simulink model "SimModelV5"  (R2021b)
settings: Solver=FixedStepAuto  StartTime=0.0  StopTime=1200  FixedStep=ts  RelTol=1e-3
InitFcn:
  | simparams
values from neighbouring files (symbols this model uses):
  A_Stirn = 2.19    [simparams.m]
  c_w = 0.25    [simparams.m]
  EngTrq = [0 25 50 75 100 125 150 175 200 225 250 275 300]    [simparams.m]
  f_roll = 0.013    [simparams.m]
  g = 9.81    [simparams.m]
  gear_1 = torque_gear1_excel    [simparams.m]
  Getriebefaktoren = [0.950000000000000	1	1.08000000000000	1.18000000000000	1.26000000000000	1.40000000000000	1.56000000000000	1.13000000000000]    [simparams.m]
  i_brems = 12    [simparams.m]
  i_GetriebeUebersetzung = [0.00, 4.31, 2.44, 1.35, 0.94, 0.82, 0.70, 3.38]    [simparams.m]
  i_UebersetzungHinterachsgetriebe = 3.35    [simparams.m]
  k_Stuetz_Pedal = [0.00 0.13 6.25 12.50 18.75 25.00 31.25 37.50 43.75 50.00 56.25 62.50 68.75 75.00 81.25 90.63 100.00]    [simparams.m]
  m_Fzg = 1525    [simparams.m]
  M_Schlepp = [10.27 10.53 10.93 11.46 12.12 12.91 13.84 14.90 16.09 17.41 18.86 20.45]    [simparams.m]
  m_Zuladung = 50    [simparams.m]
  MassefaktorenGang = [1.04, 1.32, 1.15, 1.10, 1.07, 1.06, 1.05, 1.35]    [simparams.m]
  mu_brems = 0.8    [simparams.m]
  n_brems = 2    [simparams.m]
  n_Stuetz_Motor = [0.00 608.00 640.00 736.00 800.00 992.00 1248.00 1504.00 1760.00 2016.00 2240.00 2496.00 2752.00 3008.00 3264.00 3488.00 3744.00 4000.00 4512.00 4992.00 5248.00 5500.00]    [simparams.m]
  n_Stuetz_Motor_Schlepp = [0 500 1000 1500 2000 2500 3000 3500 4000 4500 5000 5500]    [simparams.m]
  r_brems = 0.1    [simparams.m]
  r_Radradius = 0.32    [simparams.m]
  roh_air = 1.2    [simparams.m]
  torquerequeststandardcondition_pdf = [0 0 0 0 0 0 0 0 0 0 0 0 0 0 0 0 0 0 0 0 0 0 ... (first row only)    [simparams.m]
  U_Radumfang = 2*pi*r_Radradius    (= 2.0106192983)    [simparams.m]
undefined symbols (not defined in the file or in its folder): DiscIntNeverNeededParam
libraries: simulink x2, slpidlib x2
settings Model: Creator=Oli  LastModifiedBy=ruwen
settings DataIOCC: ExternalInput=[cw_drag, A_face, roh_air]

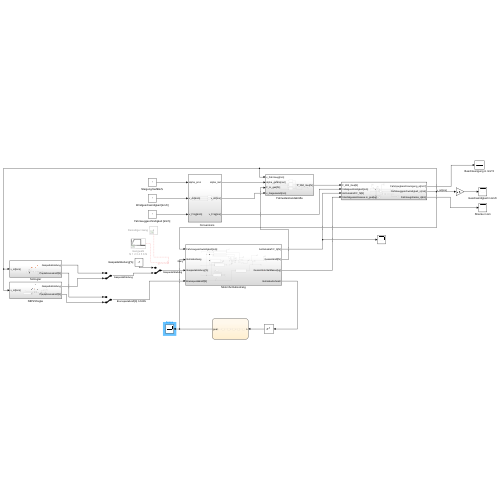
[thumbnail: Simulink's stored preview of the top-level diagram]
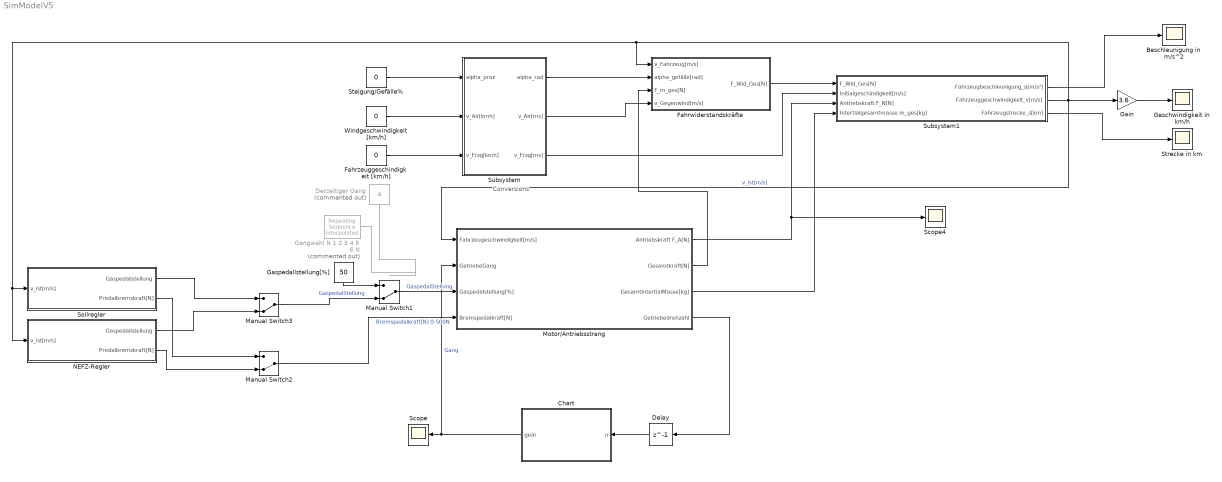
== system SimModelV5 ==
  note: Conversions
  Beschleunigung in m/s^2 : Scope
  Chart : Stateflow chart  TreatAsAtomicUnit=on
  Delay : Delay  DelayLength=1  InitialCondition=0
  Derzeitiger Gang : Constant  Commented=on  Value=4
  Fahrwiderstandskräfte : Subsystem
  Fahrzeuggeschindigkeit [km/h] : Constant  Value=0
  Gain : Gain  Gain=3.6
  Gangwahl N 1 2 3 4 5 6 N : simulink/Sources/Repeating Sequence Interpolated  Commented=on  OutValues="[0   1    2     3    4    5    6     6     0    0].'"  TimeValues=[0 100 200 300 400 500 600 2000 2001 3000].'  LookUpMeth=Use Input Below  tsamp=-1  OutMin=[]  OutMax=[]  OutDataTypeStr=double  OutputDataTypeScalingMode=double  OutDataType=fixdt(0,8)  OutScaling=2^-10
  Gaspedallstellung[%] : Constant  Value=50
  Geschwindigkeit in km/h : Scope
  Manual Switch1 : ManualSwitch  CurrentSetting=0
  Manual Switch2 : ManualSwitch  CurrentSetting=0
  Manual Switch3 : ManualSwitch  CurrentSetting=0
  Motor/Antriebsstrang : Subsystem
  NEFZ-Regler : Subsystem
  Scope : Scope
  Scope4 : Scope
  Sollregler : Subsystem
  "Steigung/Gefälle% " : Constant  Value=0
  Strecke in km : Scope
  Subsystem : Subsystem
  Subsystem1 : Subsystem
  Windgeschwindigkeit [km/h] : Constant  Value=0
  wires:
  "Steigung/Gefälle% "/1 -> Subsystem/1(alpha_proz)
  Windgeschwindigkeit [km/h]/1 -> Subsystem/2(v_Air[kmh])
  Fahrzeuggeschindigkeit [km/h]/1 -> Subsystem/3(v_Frzg[kmh])
  Subsystem/1(alpha_rad) -> Fahrwiderstandskräfte/2(alpha_gefälle[rad])
  Subsystem/2(v_Air[ms]) -> Fahrwiderstandskräfte/4(v_Gegenwind[m/s])
  Fahrwiderstandskräfte/1(F_Wid_Ges[N]) -> Subsystem1/1(F_Wid_Ges[N])
  Subsystem/3(v_Frzg[ms]) -> Subsystem1/2(Initialgeschindigkeit[m/s])
  Motor/Antriebsstrang/3(GesamtIntertialMasse[kg]) -> Subsystem1/4(Intertialgesamtmasse m_ges[kg])
  Motor/Antriebsstrang/2(Gesamtkraft[N]) -> Fahrwiderstandskräfte/3(F_m_ges[N])
  Subsystem1/3(Fahrzeugstrecke_s[km]) -> Strecke in km/1
  Subsystem1/2(Fahrzeuggeschwindigkeit_v[m/s]) -> Gain/1, Motor/Antriebsstrang/1(Fahrzeugeschwindigkeit[m/s]), NEFZ-Regler/1(v_ist[m/s]), Sollregler/1(v_ist[m/s]), Fahrwiderstandskräfte/1(v_Fahrzeug[m/s])  "v_ist[m/s]"
  Subsystem1/1(Fahrzeugbeschleunigung_a[m/s²]) -> Beschleunigung in m/s^2/1
  Derzeitiger Gang/1 -> ?
  Gangwahl N 1 2 3 4 5 6 N/1 -> ?
  Chart/1(gear) -> Motor/Antriebsstrang/2(GetriebeGang), Scope/1  "Gang"
  Gain/1 -> Geschwindigkeit in km/h/1
  Manual Switch1/1 -> Motor/Antriebsstrang/3(Gaspedalstellung[%])  "GaspedalStellung"
  Motor/Antriebsstrang/1(Antriebskraft F_A[N]) -> Subsystem1/3(Antriebskraft F_N[N]), Scope4/1
  Gaspedallstellung[%]/1 -> Manual Switch1/1
  Manual Switch2/1 -> Motor/Antriebsstrang/4(Bremspedalkraft[N])  "Bremspedalkraft[N] 0-500N"
  Manual Switch3/1 -> Manual Switch1/2  "GaspedalStellung"
  NEFZ-Regler/2(Predalbremskraft[N]) -> Manual Switch2/2
  NEFZ-Regler/1(Gaspedallstellung) -> Manual Switch3/2
  Sollregler/1(Gaspedallstellung) -> Manual Switch3/1
  Sollregler/2(Predalbremskraft[N]) -> Manual Switch2/1
  Motor/Antriebsstrang/4(Getriebedrehzahl) -> Delay/1
  Delay/1 -> Chart/1(n)

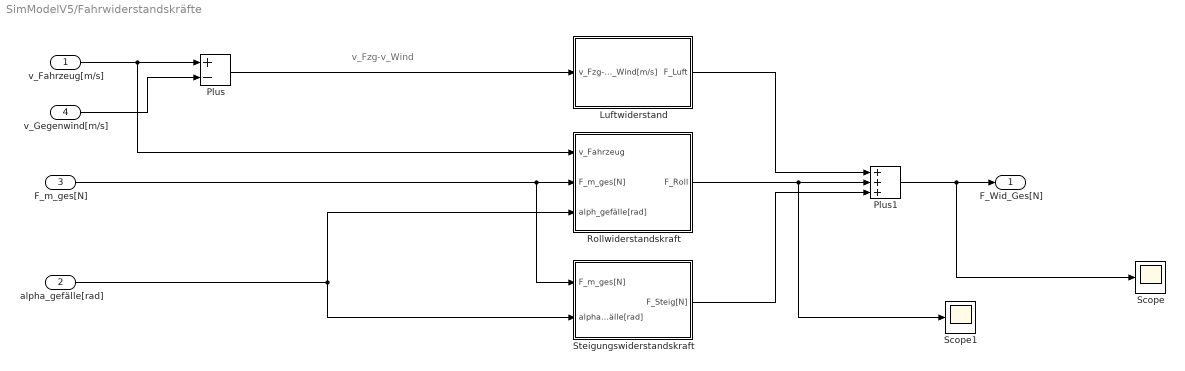
== system SimModelV5/Fahrwiderstandskräfte ==
  note: v_Fzg-v_Wind
  v_Fahrzeug[m/s] : Inport
  alpha_gefälle[rad] : Inport  Port=2
  F_m_ges[N] : Inport  Port=3
  v_Gegenwind[m/s] : Inport  Port=4
  Luftwiderstand : Subsystem
  Plus : Sum  Inputs=+-
  Plus1 : Sum  Inputs=+++
  Rollwiderstandskraft : Subsystem
  Scope : Scope
  Scope1 : Scope
  Steigungswiderstandskraft : Subsystem
  F_Wid_Ges[N] : Outport
  wires:
  v_Fahrzeug[m/s]/1 -> Rollwiderstandskraft/1(v_Fahrzeug), Plus/1
  v_Gegenwind[m/s]/1 -> Plus/2
  Plus/1 -> Luftwiderstand/1(v_Fzg-v_Wind[m/s])
  F_m_ges[N]/1 -> Steigungswiderstandskraft/1(F_m_ges[N]), Rollwiderstandskraft/2(F_m_ges[N])
  alpha_gefälle[rad]/1 -> Steigungswiderstandskraft/2(alpha_gefälle[rad]), Rollwiderstandskraft/3(alph_gefälle[rad])
  Luftwiderstand/1(F_Luft) -> Plus1/1
  Rollwiderstandskraft/1(F_Roll) -> Scope1/1, Plus1/2
  Steigungswiderstandskraft/1(F_Steig[N]) -> Plus1/3
  Plus1/1 -> F_Wid_Ges[N]/1, Scope/1

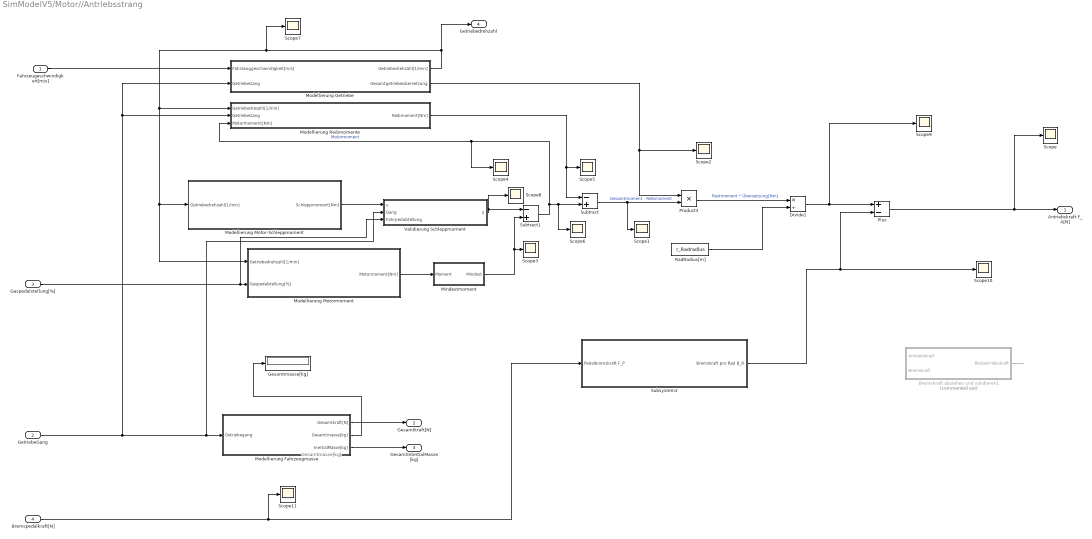
== system SimModelV5/Motor//Antriebsstrang ==
  note: Gesamtmasse[kg]
  Fahrzeugeschwindigkeit[m/s] : Inport
  GetriebeGang : Inport  Port=2
  Gaspedalstellung[%] : Inport  Port=3
  Bremspedalkraft[N] : Inport  Port=4
  Bremskraft abziehen und validieren1 : MATLAB Function  Commented=on  TreatAsAtomicUnit=on
  Divide1 : Product  Inputs=*/
  Gesamtmasse[kg] : Display
  Mindestmoment : Subsystem
  Modellierung Fahrzeugmasse : Subsystem
  Modellierung Getriebe : Subsystem
  Modellierung Motor-Schleppmoment : Subsystem
  Modellierung Motormoment : Subsystem
  Modellierung Reibmomente : Subsystem
  Plus : Sum  Inputs=+-
  Product3 : Product
  RadRadius[m] : Constant  Value=r_Radradius
  Scope{,1..11} (12 alike) : Scope
  Subsystem2 : Subsystem
  Subtract : Sum  Inputs=-+
  Subtract1 : Sum  Inputs=-+
  Validierung Schleppmoment : MATLAB Function  TreatAsAtomicUnit=on
  Antriebskraft F_A[N] : Outport
  Gesamtkraft[N] : Outport  Port=2
  GesamtIntertialMasse[kg] : Outport  Port=3
  Getriebedrehzahl : Outport  Port=4
  wires:
  GetriebeGang/1 -> Modellierung Fahrzeugmasse/1(Getriebegang), Validierung Schleppmoment/2(Gang), Modellierung Reibmomente/2(GetriebeGang), Modellierung Getriebe/2(GetriebeGang)
  Modellierung Fahrzeugmasse/1(Gesamtkraft[N]) -> Gesamtkraft[N]/1
  Modellierung Fahrzeugmasse/2(Gesamtmasse[kg]) -> Gesamtmasse[kg]/1
  Modellierung Fahrzeugmasse/3(InertialMasse[kg]) -> GesamtIntertialMasse[kg]/1
  Modellierung Getriebe/1(Getriebedrehzahl[1/min]) -> Getriebedrehzahl/1, Scope7/1, Modellierung Reibmomente/1(Getriebedrezahl[1/min]), Modellierung Motormoment/1(Getriebedrehzahl[1/min]), Modellierung Motor-Schleppmoment/1(Getriebedrehzahl[1/min])
  Fahrzeugeschwindigkeit[m/s]/1 -> Modellierung Getriebe/1(Fahrzeuggeschwindigkeit[m/s])
  Gaspedalstellung[%]/1 -> Modellierung Motormoment/2(Gaspedalstellung[%]), Validierung Schleppmoment/3(Fahrpedalstellung)
  Modellierung Motor-Schleppmoment/1(Schleppmoment[Nm]) -> Validierung Schleppmoment/1(u)
  Validierung Schleppmoment/1(y) -> Scope8/1, Subtract1/1
  Mindestmoment/1(Mindest) -> Subtract1/2, Scope3/1
  Modellierung Motormoment/1(Motormoment[Nm]) -> Mindestmoment/1(Moment)
  Subtract1/1 -> Scope6/1, Subtract/2, Scope4/1, Modellierung Reibmomente/3(Motormomemt[Nm])  "Motormoment"
  Modellierung Reibmomente/1(Reibmoment[Nm]) -> Scope5/1, Subtract/1
  Subtract/1 -> Scope1/1, Product3/2  "Gesamtmoment - Reibmoment"
  Modellierung Getriebe/2(Gesamtgetriebeübersetzung) -> Scope2/1, Product3/1
  Product3/1 -> Divide1/1  "Restmoment * Übersetzung[Nm]"
  RadRadius[m]/1 -> Divide1/2
  Divide1/1 -> Plus/1, Scope9/1
  Subsystem2/1(Bremskraft pro Rad B_R) -> Plus/2, Scope10/1
  Bremspedalkraft[N]/1 -> Scope11/1, Subsystem2/1(Pedalbremskraft F_P)
  Plus/1 -> Antriebskraft F_A[N]/1, Scope/1
  Bremskraft abziehen und validieren1/1(Restantriebskraft) -> ?

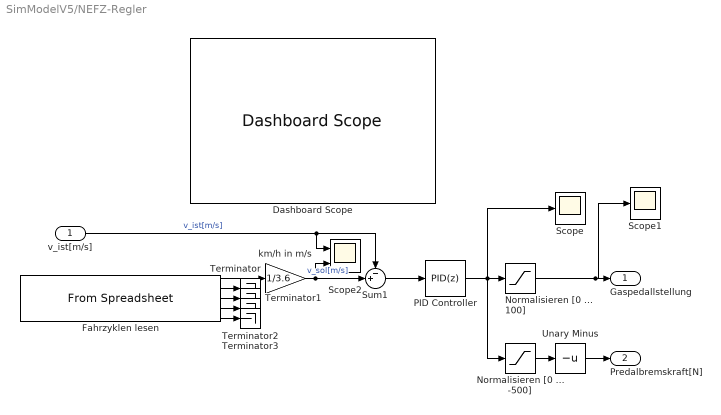
== system SimModelV5/NEFZ-Regler ==
  v_ist[m/s] : Inport
  Dashboard Scope : DashboardScope
  Fahrzyklen lesen : FromSpreadsheet  FileName=Fahrzyklen_Uebung_05.xlsx  SheetName=Tabelle1
  Normalisieren [0 ... -500] : Saturate  UpperLimit=0  LowerLimit=-500
  Normalisieren [0 ... 100] : Saturate  UpperLimit=100  LowerLimit=0
  PID Controller : slpidlib/PID Controller  Controller=PID  Form=Parallel  TimeDomain=Discrete-time  UseExternalTs=off  SampleTime=-1  IntegratorMethod=Forward Euler  FilterMethod=Forward Euler  ControllerParametersSource=internal  P=5000  I=0.78  D=0  UseFilter=on  N=100  TunerSelectOption=Transfer Function Based (PID Tuner App)  InitialConditionSource=internal  InitialConditionForIntegrator=0  InitialConditionForFilter=0  DifferentiatorICPrevScaledInput=0  ExternalReset=none  TrackingMode=off  Kt=1  LimitOutput=off  SatLimitsSource=internal  UpperSaturationLimit=inf  LowerSaturationLimit=-inf  LinearizeAsGain=on  AntiWindupMode=none  Kb=1  POutMin=[]  POutMax=[]  IOutMin=[]  IOutMax=[]  DOutMin=[]  DOutMax=[]  NOutMin=[]  NOutMax=[]  SumOutMin=[]  SumOutMax=[]  SaturationOutMin=[]  SaturationOutMax=[]  PParamMin=[]  PParamMax=[]  IParamMin=[]  IParamMax=[]  DParamMin=[]  DParamMax=[]  NParamMin=[]  NParamMax=[]  KbParamMin=[]  KbParamMax=[]  KtParamMin=[]  KtParamMax=[]  KbOutMin=[]  KbOutMax=[]  KtOutMin=[]  KtOutMax=[]  IntegratorOutMin=[]  IntegratorOutMax=[]  FilterOutMin=[]  FilterOutMax=[]  SumI1OutMin=[]  SumI1OutMax=[]  SumI2OutMin=[]  SumI2OutMax=[]  SumI3OutMin=[]  SumI3OutMax=[]  SumI4OutMin=[]  SumI4OutMax=[]  SumDOutMin=[]  SumDOutMax=[]  DifferentiatorOutMin=[]  DifferentiatorOutMax=[]  FilterDiffOutCoefMin=[]  FilterDiffOutCoefMax=[]  ReciprocalOutMin=[]  ReciprocalOutMax=[]  SumDenOutMin=[]  SumDenOutMax=[]  SumNumOutMin=[]  SumNumOutMax=[]  DivideOutMin=[]  DivideOutMax=[]  UdiffTsProdOutMin=[]  UdiffTsProdOutMax=[]  NTsProdOutMin=[]  NTsProdOutMax=[]  UintegralTsProdOutMin=[]  UintegralTsProdOutMax=[]  UngainTsProdOutMin=[]  UngainTsProdOutMax=[]  IntegratorContinuousStateAttributes=''  IntegratorStateMustResolveToSignalObject=off  IntegratorRTWStateStorageClass=Auto  FilterContinuousStateAttributes=''  FilterStateMustResolveToSignalObject=off  FilterRTWStateStorageClass=Auto  ParallelPVariant=InternalParameters  IdealPVariant=Disabled  IVariant=InternalParameters  DVariant=InternalParameters  IntegratorVariant=Discrete  SatVariant=Disabled  AWVariant=Passthrough  PCopyVariant=Disabled  TRVariant=Disabled  FdbkBlocksVariant=Forward  IdealPFdbkVariant=Disabled  SatFdbkVariant=Disabled  DerivativeFilterVariant=ForwardEulerFilter  NVariant=InternalParameters  NCopyVariant=Disabled  FilterICVariant=InternalICsFilter  IntegratorICVariant=InternalICs  ExternalResetVariant=Disabled  TRSumVariant=Passthrough  SumFdbkVariant=Disabled  SumVariant=Sum_PID  TsampFilterVariant=InternalTs  TsampNgainVariant=Passthrough  TsampIntegralVariant=Passthrough  ExternalSaturationOutDataTypeStr=Inherit: Same as second input
  Scope : Scope
  Scope1 : Scope
  Scope2 : Scope  NumInputPorts=2
  Sum1 : Sum  Inputs=-+|
  Terminator{,1..3} (4 alike) : Terminator
  Unary Minus : UnaryMinus
  km/h in m/s : Gain  Gain=1/3.6
  Gaspedallstellung : Outport
  Predalbremskraft[N] : Outport  Port=2
  wires:
  km/h in m/s/1 -> Sum1/2, Scope2/2  "v_sol[m/s]"
  Sum1/1 -> PID Controller/1
  v_ist[m/s]/1 -> Scope2/1, Sum1/1  "v_ist[m/s]"
  PID Controller/1 -> Scope/1, Normalisieren [0 ... -500]/1, Normalisieren [0 ... 100]/1
  Normalisieren [0 ... 100]/1 -> Scope1/1, Gaspedallstellung/1
  Fahrzyklen lesen/2 -> Terminator/1
  Fahrzyklen lesen/3 -> Terminator1/1
  Fahrzyklen lesen/4 -> Terminator2/1
  Fahrzyklen lesen/5 -> Terminator3/1
  Fahrzyklen lesen/1 -> km/h in m/s/1
  Normalisieren [0 ... -500]/1 -> Unary Minus/1
  Unary Minus/1 -> Predalbremskraft[N]/1

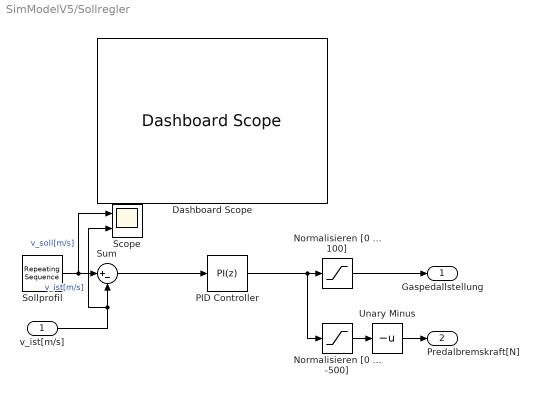
== system SimModelV5/Sollregler ==
  v_ist[m/s] : Inport
  Dashboard Scope : DashboardScope
  Normalisieren [0 ... -500] : Saturate  UpperLimit=0  LowerLimit=-500
  Normalisieren [0 ... 100] : Saturate  UpperLimit=100  LowerLimit=0
  PID Controller : slpidlib/PID Controller  Controller=PI  Form=Parallel  TimeDomain=Discrete-time  UseExternalTs=off  SampleTime=-1  IntegratorMethod=Forward Euler  FilterMethod=Forward Euler  ControllerParametersSource=internal  P=25  I=1  D=-1  UseFilter=on  N=100  TunerSelectOption=Transfer Function Based (PID Tuner App)  InitialConditionSource=internal  InitialConditionForIntegrator=0  InitialConditionForFilter=0  DifferentiatorICPrevScaledInput=0  ExternalReset=none  TrackingMode=off  Kt=1  LimitOutput=off  SatLimitsSource=internal  UpperSaturationLimit=inf  LowerSaturationLimit=-inf  LinearizeAsGain=on  AntiWindupMode=none  Kb=1  POutMin=[]  POutMax=[]  IOutMin=[]  IOutMax=[]  DOutMin=[]  DOutMax=[]  NOutMin=[]  NOutMax=[]  SumOutMin=[]  SumOutMax=[]  SaturationOutMin=[]  SaturationOutMax=[]  PParamMin=[]  PParamMax=[]  IParamMin=[]  IParamMax=[]  DParamMin=[]  DParamMax=[]  NParamMin=[]  NParamMax=[]  KbParamMin=[]  KbParamMax=[]  KtParamMin=[]  KtParamMax=[]  KbOutMin=[]  KbOutMax=[]  KtOutMin=[]  KtOutMax=[]  IntegratorOutMin=[]  IntegratorOutMax=[]  FilterOutMin=[]  FilterOutMax=[]  SumI1OutMin=[]  SumI1OutMax=[]  SumI2OutMin=[]  SumI2OutMax=[]  SumI3OutMin=[]  SumI3OutMax=[]  SumI4OutMin=[]  SumI4OutMax=[]  SumDOutMin=[]  SumDOutMax=[]  DifferentiatorOutMin=[]  DifferentiatorOutMax=[]  FilterDiffOutCoefMin=[]  FilterDiffOutCoefMax=[]  ReciprocalOutMin=[]  ReciprocalOutMax=[]  SumDenOutMin=[]  SumDenOutMax=[]  SumNumOutMin=[]  SumNumOutMax=[]  DivideOutMin=[]  DivideOutMax=[]  UdiffTsProdOutMin=[]  UdiffTsProdOutMax=[]  NTsProdOutMin=[]  NTsProdOutMax=[]  UintegralTsProdOutMin=[]  UintegralTsProdOutMax=[]  UngainTsProdOutMin=[]  UngainTsProdOutMax=[]  IntegratorContinuousStateAttributes=''  IntegratorStateMustResolveToSignalObject=off  IntegratorRTWStateStorageClass=Auto  FilterContinuousStateAttributes=''  FilterStateMustResolveToSignalObject=off  FilterRTWStateStorageClass=Auto  ParallelPVariant=InternalParameters  IdealPVariant=Disabled  IVariant=InternalParameters  DVariant=Disabled  IntegratorVariant=Discrete  SatVariant=Disabled  AWVariant=Passthrough  PCopyVariant=Disabled  TRVariant=Disabled  FdbkBlocksVariant=Forward  IdealPFdbkVariant=Disabled  SatFdbkVariant=Disabled  DerivativeFilterVariant=Disabled  NVariant=Disabled  NCopyVariant=Disabled_SignalSpec  FilterICVariant=Disabled  IntegratorICVariant=InternalICs  ExternalResetVariant=Disabled  TRSumVariant=Passthrough  SumFdbkVariant=Disabled  SumVariant=Sum_PI  TsampFilterVariant=InternalTs  TsampNgainVariant=Passthrough  TsampIntegralVariant=Passthrough  ExternalSaturationOutDataTypeStr=Inherit: Same as second input
  Scope : Scope  NumInputPorts=2
  Sollprofil : simulink/Sources/Repeating Sequence  rep_seq_t=[0 50 100 1100 1150 1200]  rep_seq_y=[0 0 27 44 0 0]
  Sum : Sum  Inputs=|+-
  Unary Minus : UnaryMinus
  Gaspedallstellung : Outport
  Predalbremskraft[N] : Outport  Port=2
  wires:
  Sollprofil/1 -> Scope/1, Sum/1  "v_soll[m/s]"
  v_ist[m/s]/1 -> Scope/2, Sum/2  "v_ist[m/s]"
  PID Controller/1 -> Normalisieren [0 ... -500]/1, Normalisieren [0 ... 100]/1
  Normalisieren [0 ... 100]/1 -> Gaspedallstellung/1
  Sum/1 -> PID Controller/1
  Normalisieren [0 ... -500]/1 -> Unary Minus/1
  Unary Minus/1 -> Predalbremskraft[N]/1

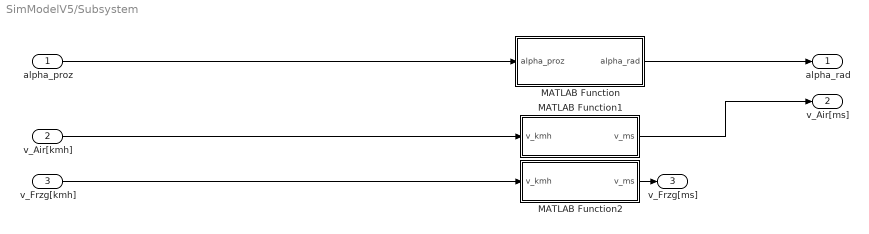
== system SimModelV5/Subsystem ==
  alpha_proz : Inport
  v_Air[kmh] : Inport  Port=2
  v_Frzg[kmh] : Inport  Port=3
  MATLAB Function : MATLAB Function  TreatAsAtomicUnit=on
  MATLAB Function1 : MATLAB Function  TreatAsAtomicUnit=on
  MATLAB Function2 : MATLAB Function  TreatAsAtomicUnit=on
  alpha_rad : Outport
  v_Air[ms] : Outport  Port=2
  v_Frzg[ms] : Outport  Port=3
  wires:
  v_Frzg[kmh]/1 -> MATLAB Function2/1(v_kmh)
  MATLAB Function/1(alpha_rad) -> alpha_rad/1
  alpha_proz/1 -> MATLAB Function/1(alpha_proz)
  MATLAB Function2/1(v_ms) -> v_Frzg[ms]/1
  v_Air[kmh]/1 -> MATLAB Function1/1(v_kmh)
  MATLAB Function1/1(v_ms) -> v_Air[ms]/1

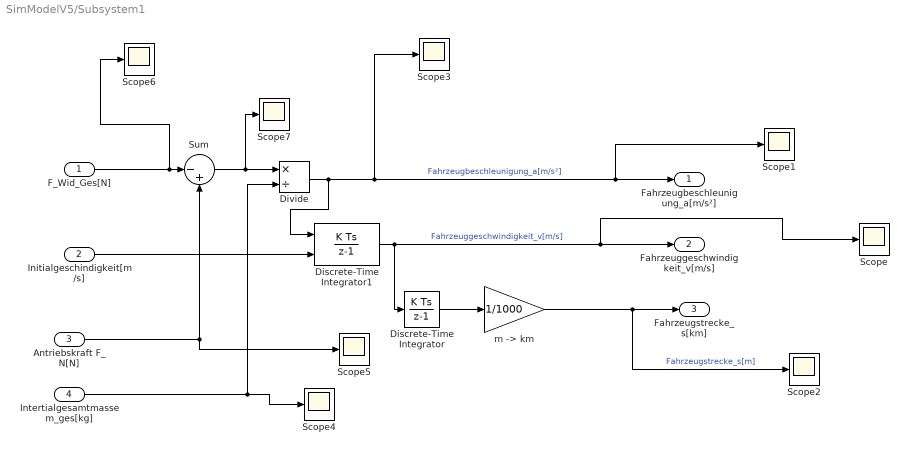
== system SimModelV5/Subsystem1 ==
  F_Wid_Ges[N] : Inport
  Initialgeschindigkeit[m/s] : Inport  Port=2
  Antriebskraft F_N[N] : Inport  Port=3
  Intertialgesamtmasse m_ges[kg] : Inport  Port=4
  Discrete-Time Integrator : DiscreteIntegrator  SampleTime=-1  ICPrevOutput=DiscIntNeverNeededParam  ICPrevScaledInput=DiscIntNeverNeededParam
  Discrete-Time Integrator1 : DiscreteIntegrator  InitialConditionSource=external  SampleTime=-1  LimitOutput=on  UpperSaturationLimit=100  ICPrevOutput=DiscIntNeverNeededParam  ICPrevScaledInput=DiscIntNeverNeededParam
  Divide : Product  Inputs=*/
  Scope{,1..7} (8 alike) : Scope
  Sum : Sum  Inputs=|-+
  "m -> km" : Gain  Gain=1/1000
  Fahrzeugbeschleunigung_a[m/s²] : Outport
  Fahrzeuggeschwindigkeit_v[m/s] : Outport  Port=2
  Fahrzeugstrecke_s[km] : Outport  Port=3
  wires:
  Sum/1 -> Scope7/1, Divide/1
  "m -> km"/1 -> Scope2/1, Fahrzeugstrecke_s[km]/1  "Fahrzeugstrecke_s[m]"
  Divide/1 -> Discrete-Time Integrator1/1, Scope3/1, Scope1/1, Fahrzeugbeschleunigung_a[m/s²]/1  "Fahrzeugbeschleunigung_a[m/s²]"
  Discrete-Time Integrator/1 -> "m -> km"/1
  Intertialgesamtmasse m_ges[kg]/1 -> Scope4/1, Divide/2
  F_Wid_Ges[N]/1 -> Scope6/1, Sum/1
  Discrete-Time Integrator1/1 -> Discrete-Time Integrator/1, Scope/1, Fahrzeuggeschwindigkeit_v[m/s]/1  "Fahrzeuggeschwindigkeit_v[m/s]"
  Antriebskraft F_N[N]/1 -> Scope5/1, Sum/2
  Initialgeschindigkeit[m/s]/1 -> Discrete-Time Integrator1/2

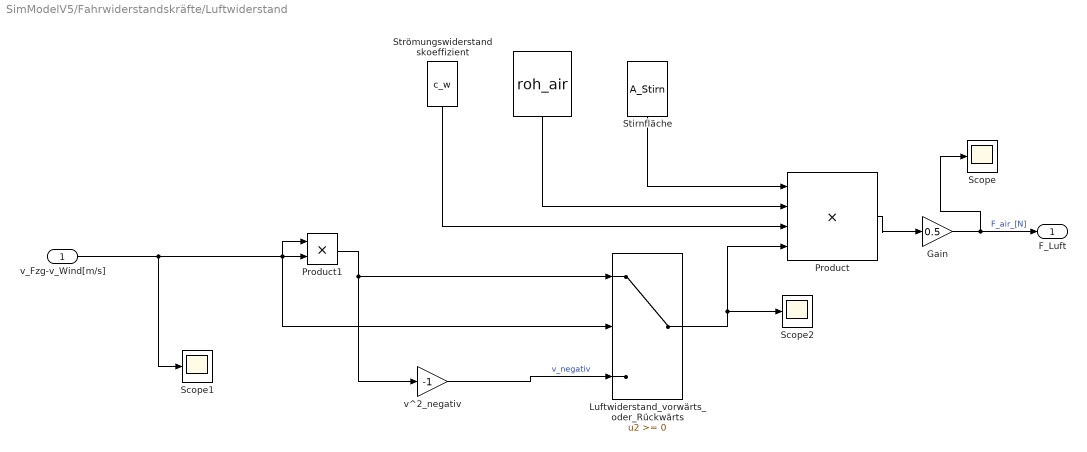
== system SimModelV5/Fahrwiderstandskräfte/Luftwiderstand ==
  v_Fzg-v_Wind[m/s] : Inport
  " " : Constant  Value=roh_air
  Gain : Gain  Gain=0.5
  Luftwiderstand_vorwärts_oder_Rückwärts : Switch
  Product : Product  Inputs=4
  Product1 : Product
  Scope : Scope
  Scope1 : Scope
  Scope2 : Scope
  Stirnfläche : Constant  Value=A_Stirn
  Strömungswiderstandskoeffizient : Constant  Value=c_w
  v^2_negativ : Gain  Gain=-1
  F_Luft : Outport
  wires:
  v_Fzg-v_Wind[m/s]/1 -> Luftwiderstand_vorwärts_oder_Rückwärts/2, Product1/2, Product1/1, Scope1/1
  Strömungswiderstandskoeffizient/1 -> Product/3
  " "/1 -> Product/2
  Stirnfläche/1 -> Product/1
  Product/1 -> Gain/1
  Product1/1 -> v^2_negativ/1, Luftwiderstand_vorwärts_oder_Rückwärts/1
  v^2_negativ/1 -> Luftwiderstand_vorwärts_oder_Rückwärts/3  "v_negativ"
  Luftwiderstand_vorwärts_oder_Rückwärts/1 -> Scope2/1, Product/4
  Gain/1 -> Scope/1, F_Luft/1  "F_air_[N]"

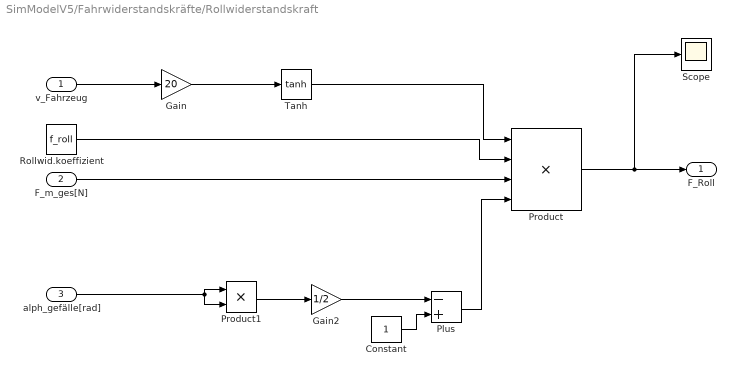
== system SimModelV5/Fahrwiderstandskräfte/Rollwiderstandskraft ==
  v_Fahrzeug : Inport
  F_m_ges[N] : Inport  Port=2
  alph_gefälle[rad] : Inport  Port=3
  Constant : Constant
  Gain : Gain  Gain=20
  Gain2 : Gain  Gain=1/2
  Plus : Sum  Inputs=-+
  Product : Product  Inputs=4
  Product1 : Product
  Rollwid.koeffizient : Constant  Value=f_roll
  Scope : Scope
  Tanh : Trigonometry  Operator=tanh
  F_Roll : Outport
  wires:
  v_Fahrzeug/1 -> Gain/1
  Product/1 -> Scope/1, F_Roll/1
  Gain2/1 -> Plus/1
  Product1/1 -> Gain2/1
  alph_gefälle[rad]/1 -> Product1/1, Product1/2
  Constant/1 -> Plus/2
  Plus/1 -> Product/4
  F_m_ges[N]/1 -> Product/3
  Gain/1 -> Tanh/1
  Rollwid.koeffizient/1 -> Product/2
  Tanh/1 -> Product/1

== system SimModelV5/Fahrwiderstandskräfte/Steigungswiderstandskraft ==
  F_m_ges[N] : Inport
  alpha_gefälle[rad] : Inport  Port=2
  Cos1 : Trigonometry
  Product2 : Product
  F_Steig[N] : Outport
  wires:
  F_m_ges[N]/1 -> Product2/1
  Cos1/1 -> Product2/2
  Product2/1 -> F_Steig[N]/1
  alpha_gefälle[rad]/1 -> Cos1/1

== system SimModelV5/Motor//Antriebsstrang/Mindestmoment ==
  Moment : Inport
  Constant : Constant  Value=0
  GreaterThanOrEqual : RelationalOperator  OutDataTypeStr=boolean  RndMeth=Simplest
  Product1 : Product
  Mindest : Outport
  wires:
  GreaterThanOrEqual/1 -> Product1/2
  Moment/1 -> GreaterThanOrEqual/1, Product1/1
  Product1/1 -> Mindest/1
  Constant/1 -> GreaterThanOrEqual/2

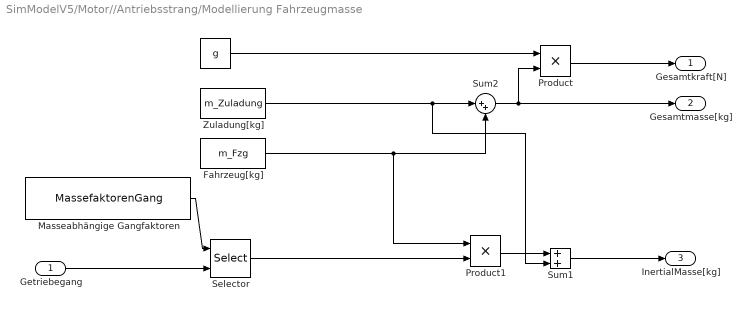
== system SimModelV5/Motor//Antriebsstrang/Modellierung Fahrzeugmasse ==
  Getriebegang : Inport
  " " : Constant  Value=g
  Fahrzeug[kg] : Constant  Value=m_Fzg
  Masseabhängige Gangfaktoren : Constant  Value=MassefaktorenGang
  Product : Product
  Product1 : Product
  Selector : Selector  IndexMode=Zero-based  InputPortWidth=8  IndexOptions=Index vector (port)  Indices=[1 3]  OutputSizes=1
  Sum1 : Sum  Inputs=++|
  Sum2 : Sum  Inputs=|++
  Zuladung[kg] : Constant  Value=m_Zuladung
  Gesamtkraft[N] : Outport
  Gesamtmasse[kg] : Outport  Port=2
  InertialMasse[kg] : Outport  Port=3
  wires:
  Sum2/1 -> Gesamtmasse[kg]/1, Product/2
  Zuladung[kg]/1 -> Sum1/2, Sum2/1
  Product/1 -> Gesamtkraft[N]/1
  " "/1 -> Product/1
  Fahrzeug[kg]/1 -> Product1/1, Sum2/2
  Getriebegang/1 -> Selector/2
  Masseabhängige Gangfaktoren/1 -> Selector/1
  Selector/1 -> Product1/2
  Product1/1 -> Sum1/1
  Sum1/1 -> InertialMasse[kg]/1

== system SimModelV5/Motor//Antriebsstrang/Modellierung Getriebe ==
  Fahrzeuggeschwindigkeit[m/s] : Inport
  GetriebeGang : Inport  Port=2
  Drehzahl : Subsystem
  Übersetzung : Subsystem
  Getriebedrehzahl[1/min] : Outport
  Gesamtgetriebeübersetzung : Outport  Port=2
  wires:
  Übersetzung/1(Gesamtübersetzung) -> Drehzahl/2(i_ges), Gesamtgetriebeübersetzung/1
  GetriebeGang/1 -> Übersetzung/1(Gang)
  Fahrzeuggeschwindigkeit[m/s]/1 -> Drehzahl/1(v)
  Drehzahl/1(n) -> Getriebedrehzahl[1/min]/1

== system SimModelV5/Motor//Antriebsstrang/Modellierung Motor-Schleppmoment ==
  Getriebedrehzahl[1/min] : Inport
  Interpolation Using Prelookup : Interpolation_n-D  NumberOfTableDimensions=1  TableSource=Input port  InternalRulePriority=Speed
      settings: InputPortMap=u0,u1,p2
  Prelookup : PreLookup  BreakpointsDataSource=Input port  BreakpointsData=[10:10:110]  BeginIndexSearchUsingPreviousIndexResult=on  ExtrapMethod=Linear
      settings: InputPortMap=u0,p1
  Schleppmoment[N] : Constant  Value=M_Schlepp
  Scope : Scope
  Stützstelle Motordrehzahl : Constant  Value=n_Stuetz_Motor_Schlepp
  Schleppmoment[Nm] : Outport
  wires:
  Getriebedrehzahl[1/min]/1 -> Prelookup/1
  Stützstelle Motordrehzahl/1 -> Prelookup/2
  Prelookup/2 -> Interpolation Using Prelookup/2
  Prelookup/1 -> Interpolation Using Prelookup/1
  Schleppmoment[N]/1 -> Interpolation Using Prelookup/3
  Interpolation Using Prelookup/1 -> Scope/1, Schleppmoment[Nm]/1

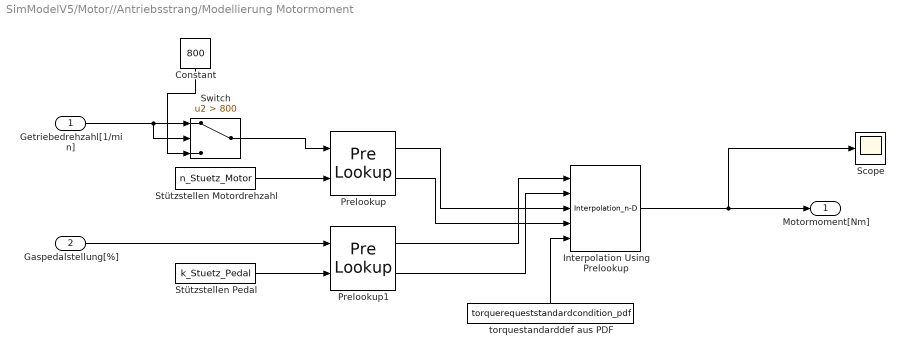
== system SimModelV5/Motor//Antriebsstrang/Modellierung Motormoment ==
  Getriebedrehzahl[1/min] : Inport
  Gaspedalstellung[%] : Inport  Port=2
  Constant : Constant  Value=800
  Interpolation Using Prelookup : Interpolation_n-D  TableSource=Input port  InternalRulePriority=Speed
      settings: InputPortMap=u0,u1,u2,u3,p2
  Prelookup : PreLookup  BreakpointsDataSource=Input port  BreakpointsData=[10:10:110]  BeginIndexSearchUsingPreviousIndexResult=on  ExtrapMethod=Linear
      settings: InputPortMap=u0,p1
  Prelookup1 : PreLookup  BreakpointsDataSource=Input port  BreakpointsData=[10:10:110]  BeginIndexSearchUsingPreviousIndexResult=on  ExtrapMethod=Linear
      settings: InputPortMap=u0,p1
  Scope : Scope
  Stützstellen Motordrehzahl : Constant  Value=n_Stuetz_Motor
  Stützstellen Pedal : Constant  Value=k_Stuetz_Pedal
  Switch : Switch  Criteria=u2 > Threshold  Threshold=800
  torquestandarddef aus PDF : Constant  Value=torquerequeststandardcondition_pdf
  Motormoment[Nm] : Outport
  wires:
  Getriebedrehzahl[1/min]/1 -> Switch/2, Switch/1
  Constant/1 -> Switch/3
  Switch/1 -> Prelookup/1
  Stützstellen Motordrehzahl/1 -> Prelookup/2
  Gaspedalstellung[%]/1 -> Prelookup1/1
  Stützstellen Pedal/1 -> Prelookup1/2
  Prelookup1/1 -> Interpolation Using Prelookup/1
  Prelookup1/2 -> Interpolation Using Prelookup/2
  Prelookup/1 -> Interpolation Using Prelookup/3
  Prelookup/2 -> Interpolation Using Prelookup/4
  torquestandarddef aus PDF/1 -> Interpolation Using Prelookup/5
  Interpolation Using Prelookup/1 -> Scope/1, Motormoment[Nm]/1

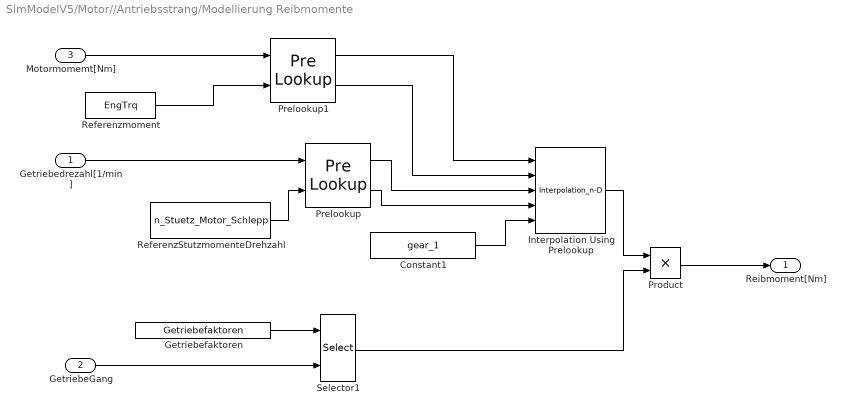
== system SimModelV5/Motor//Antriebsstrang/Modellierung Reibmomente ==
  Getriebedrezahl[1/min] : Inport
  GetriebeGang : Inport  Port=2
  Motormomemt[Nm] : Inport  Port=3
  Constant1 : Constant  Value=gear_1
  Getriebefaktoren : Constant  Value=Getriebefaktoren
  Interpolation Using Prelookup : Interpolation_n-D  TableSource=Input port  InternalRulePriority=Speed
      settings: InputPortMap=u0,u1,u2,u3,p2
  Prelookup : PreLookup  BreakpointsDataSource=Input port  BreakpointsData=[10:10:110]  BeginIndexSearchUsingPreviousIndexResult=on  ExtrapMethod=Linear
      settings: InputPortMap=u0,p1
  Prelookup1 : PreLookup  BreakpointsDataSource=Input port  BreakpointsData=[10:10:110]  BeginIndexSearchUsingPreviousIndexResult=on  ExtrapMethod=Linear
      settings: InputPortMap=u0,p1
  Product : Product
  ReferenzStutzmomenteDrehzahl : Constant  Value=n_Stuetz_Motor_Schlepp
  Referenzmoment : Constant  Value=EngTrq
  Selector1 : Selector  IndexMode=Zero-based  InputPortWidth=8  IndexOptions=Index vector (port)  Indices=[1 3]  OutputSizes=1
  Reibmoment[Nm] : Outport
  wires:
  Getriebedrezahl[1/min]/1 -> Prelookup/1
  ReferenzStutzmomenteDrehzahl/1 -> Prelookup/2
  Motormomemt[Nm]/1 -> Prelookup1/1
  Referenzmoment/1 -> Prelookup1/2
  GetriebeGang/1 -> Selector1/2
  Getriebefaktoren/1 -> Selector1/1
  Constant1/1 -> Interpolation Using Prelookup/5
  Prelookup1/1 -> Interpolation Using Prelookup/1
  Prelookup1/2 -> Interpolation Using Prelookup/2
  Prelookup/1 -> Interpolation Using Prelookup/3
  Prelookup/2 -> Interpolation Using Prelookup/4
  Interpolation Using Prelookup/1 -> Product/1
  Product/1 -> Reibmoment[Nm]/1
  Selector1/1 -> Product/2

== system SimModelV5/Motor//Antriebsstrang/Subsystem2 ==
  Pedalbremskraft F_P : Inport
  " " : Constant  Value=n_brems
  Constant5 : Constant  Value=r_brems
  Constant6 : Constant  Value=r_Radradius
  Constant7 : Constant  Value=mu_brems
  Constant9 : Constant  Value=i_brems
  Radbremskraft-Berechnung : MATLAB Function  TreatAsAtomicUnit=on
  Bremskraft pro Rad B_R : Outport
  wires:
  Constant5/1 -> Radbremskraft-Berechnung/1(r_w)
  Constant6/1 -> Radbremskraft-Berechnung/2(r_dyn)
  Constant7/1 -> Radbremskraft-Berechnung/3(mu)
  " "/1 -> Radbremskraft-Berechnung/4(n)
  Constant9/1 -> Radbremskraft-Berechnung/5(i_b)
  Pedalbremskraft F_P/1 -> Radbremskraft-Berechnung/6(F_P)
  Radbremskraft-Berechnung/1(F_BR) -> Bremskraft pro Rad B_R/1

== system SimModelV5/Motor//Antriebsstrang/Modellierung Getriebe/Drehzahl ==
  v : Inport
  i_ges : Inport  Port=2
  " " : Constant  Value=U_Radumfang
  Divide : Product  Inputs=/*
  Product1 : Product
  Umwandlung zu 1/min : Gain  Gain=60
  n : Outport
  wires:
  Divide/1 -> Product1/1
  Product1/1 -> Umwandlung zu 1/min/1
  i_ges/1 -> Product1/2
  " "/1 -> Divide/1
  v/1 -> Divide/2
  Umwandlung zu 1/min/1 -> n/1

== system SimModelV5/Motor//Antriebsstrang/Modellierung Getriebe/Übersetzung ==
  Gang : Inport
  Getriebeübersetzung1 : Constant  Value=i_GetriebeUebersetzung
  Hinterachsübersetzung : Constant  Value=i_UebersetzungHinterachsgetriebe
  Product : Product
  Selector1 : Selector  IndexMode=Zero-based  InputPortWidth=8  IndexOptions=Index vector (port)  Indices=[1 3]  OutputSizes=1
  Gesamtübersetzung : Outport
  wires:
  Getriebeübersetzung1/1 -> Selector1/1
  Gang/1 -> Selector1/2
  Hinterachsübersetzung/1 -> Product/1
  Selector1/1 -> Product/2
  Product/1 -> Gesamtübersetzung/1

== matlab function SimModelV5/Subsystem/MATLAB Function1 ==
  data: v_kmh input; v_ms output
function v_ms = kmh_to_ms(v_kmh)

v_ms = v_kmh/3.6;

== matlab function SimModelV5/Subsystem/MATLAB Function ==
  data: alpha_proz input; alpha_rad output
function alpha_rad = steigProzToRad(alpha_proz)

alpha_rad = atan(alpha_proz/100);

== matlab function SimModelV5/Subsystem/MATLAB Function2 ==
  data: v_kmh input; v_ms output
function v_ms = kmh_to_ms(v_kmh)

v_ms = v_kmh/3.6;

== matlab function SimModelV5/Motor//Antriebsstrang/Validierung Schleppmoment ==
  data: u input; y output; Gang input; Fahrpedalstellung input
%Validierung des Schleppmoments: Wenn der Neutralgang eingelegt ist oder wenn die 
%Fahrpedalstellung >0 ist soll das Schleppmoment nicht wirken.

function y = fcn(u, Gang, Fahrpedalstellung)

if Gang == 0 || Fahrpedalstellung>0
    y=0;
else
    y=u;
end

== matlab function SimModelV5/Motor//Antriebsstrang/Bremskraft abziehen und validieren1 ==
  data: Antriebskraft input; Restantriebskraft output; Bremskraft input
function Restantriebskraft = fcn(Antriebskraft, Bremskraft)

    if Bremskraft>=Antriebskraft
        Restantriebskraft = 0;
    else
        Restantriebskraft = Antriebskraft + Bremskraft;
    end

== matlab function SimModelV5/Motor//Antriebsstrang/Subsystem2/Radbremskraft-Berechnung ==
  data: r_w input; F_BR output; r_dyn input; mu input; n input; i_b input; F_P input
function F_BR = fcn(r_w, r_dyn, mu, n, i_b, F_P)


F_BR = (r_w/r_dyn) * mu * n * i_b * F_P;

== stateflow chart SimModelV5/Chart ==
  state GEAR_1
    entry:
    gear = 1;
  state GEAR_2
    entry:
    gear = 2;
  state GEAR_3
    entry:
    gear = 3;
  state GEAR_4
    entry:
    gear = 4;
  state GEAR_5
    entry:
    gear = 5;
  state GEAR_6
    entry:
    gear = 6;
  (default) -> GEAR_1
  GEAR_1 -> GEAR_2 : [n>3500]
  GEAR_2 -> GEAR_3 [order 1] : [n>3500]
  GEAR_3 -> GEAR_4 [order 1] : [n>3500]
  GEAR_5 -> GEAR_6 [order 1] : [n>3500]
  GEAR_4 -> GEAR_5 [order 1] : [n>3500]
  GEAR_6 -> GEAR_5 : [n<1500]
  GEAR_5 -> GEAR_4 [order 2] : [n<1500]
  GEAR_3 -> GEAR_2 [order 2] : [n<1500]
  GEAR_4 -> GEAR_3 [order 2] : [n<1500]
  GEAR_2 -> GEAR_1 [order 2] : [n<1500]
  data: n input; gear output
